simulink model "ControlBA"  (R2022b)
settings: Solver=VariableStepAuto  StartTime=0.0  StopTime=10.0  RelTol=1e-3
settings Model: Creator=David  LastModifiedBy=Usuario

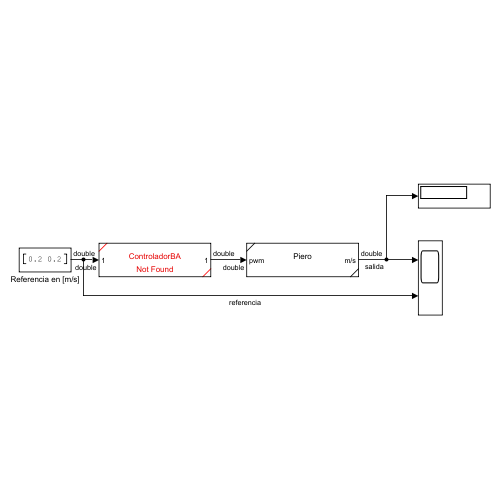
[thumbnail: Simulink's stored preview of the top-level diagram]
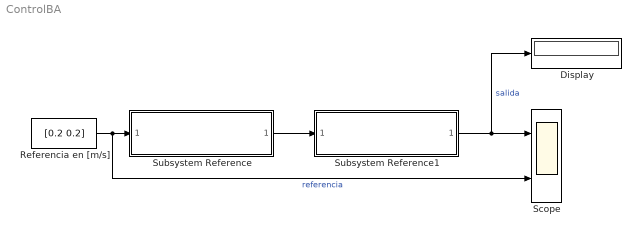
== system ControlBA ==
  Display : Display
  Referencia en [m/s] : Constant  Value=[0.2 0.2]
  Scope : Scope  NumInputPorts=2
  Subsystem Reference : Subsystem  ReferencedSubsystem=ControladorBA
  Subsystem Reference1 : Subsystem  ReferencedSubsystem=Piero
  wires:
  Subsystem Reference/1 -> Subsystem Reference1/1
  Referencia en [m/s]/1 -> Scope/2, Subsystem Reference/1  "referencia"
  Subsystem Reference1/1 -> Display/1, Scope/1  "salida"
